simulink model "motorcontrol_19a_v2"  (R2019b)
settings: Solver=FixedStepDiscrete  StartTime=0.0  StopTime=Inf  FixedStep=Ts.pwm  MaxStep=5e-5  RelTol=1e-3  EnableMultiTasking=on
undefined symbols (not defined in the file): ControlMode, ctrlParams, dataType, DiscIntNeverNeededParam, Down, GPTRIP1SEL, GPTRIP2SEL, inverter, mcb_isSimVar, NumBits1, NumBits2, PI_params, pmsm, Slope1, Slope2, Target, Ts, TZ1, TZ2, Up
libraries: simulink x14, c2802xlib x7, c2837xDlib x3, c280xlib x1, c2000lib x1
(part 3 of 3)

== system motorcontrol_19a_v2/Motor_Control1/ControlSystem/Closed_Loop/Current_Controllers/FeedForward Decoupling Compensation ==
  d_current measured : Inport
  Electrical_speed measured : Inport  Port=2
  q_current measured : Inport  Port=3
  Add : Sum
  Constant : Constant  Value=pmsm.Ld  OutDataTypeStr=Inherit: Inherit via back propagation  SampleTime=-1
  Constant1 : Constant  Value=pmsm.FluxPM  OutDataTypeStr=Inherit: Inherit via back propagation  SampleTime=-1
  Constant2 : Constant  Value=pmsm.Lq  OutDataTypeStr=Inherit: Inherit via back propagation  SampleTime=-1
  Data Type Duplicate : DataTypeDuplicate  NumInputPorts=6
  Product4 : Product  Inputs=3
  Product5 : Product
  Product6 : Product
  Unary Minus : UnaryMinus
  q_voltage_compensation : Outport
  d_voltage_compensation : Outport  Port=2
  wires:
  q_current measured/1 -> Product4/2, Data Type Duplicate/1
  Constant1/1 -> Data Type Duplicate/5, Add/2
  Product6/1 -> d_voltage_compensation/1
  Product4/1 -> Unary Minus/1
  Unary Minus/1 -> q_voltage_compensation/1
  Constant/1 -> Data Type Duplicate/4, Product5/2
  Product5/1 -> Add/1
  Electrical_speed measured/1 -> Product4/3, Product6/1, Data Type Duplicate/2
  Add/1 -> Product6/2
  d_current measured/1 -> Product5/1, Data Type Duplicate/3
  Constant2/1 -> Product4/1, Data Type Duplicate/6

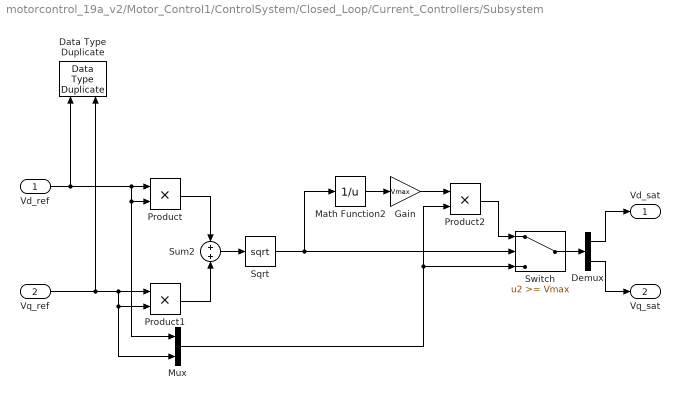
== system motorcontrol_19a_v2/Motor_Control1/ControlSystem/Closed_Loop/Current_Controllers/Subsystem ==
  Vd_ref : Inport
  Vq_ref : Inport  Port=2
  Data Type Duplicate : DataTypeDuplicate
  Demux : Demux  Outputs=2
  Gain : Gain  Gain=Vmax  OutDataTypeStr=Inherit: Same as input
  Math Function2 : Math  Operator=reciprocal  RndMeth=Simplest
  Mux : Mux  Inputs=2
  Product : Product  RndMeth=Simplest  OutDataTypeStr=Inherit: Same as first input
  Product1 : Product  RndMeth=Simplest  OutDataTypeStr=Inherit: Same as first input
  Product2 : Product  OutDataTypeStr=Inherit: Same as first input
  Sqrt : Sqrt  IntermediateResultsDataTypeStr=Inherit: Inherit from input  SaturateOnIntegerOverflow=on
  Sum2 : Sum  OutDataTypeStr=Inherit: Same as first input
  Switch : Switch  Threshold=Vmax  ZeroCross=off
  Vd_sat : Outport  VectorParamsAs1DForOutWhenUnconnected=off
  Vq_sat : Outport  Port=2  VectorParamsAs1DForOutWhenUnconnected=off
  wires:
  Vd_ref/1 -> Mux/1, Product/2, Product/1, Data Type Duplicate/1
  Demux/1 -> Vd_sat/1
  Product1/1 -> Sum2/2
  Product/1 -> Sum2/1
  Sum2/1 -> Sqrt/1
  Gain/1 -> Product2/1
  Math Function2/1 -> Gain/1
  Vq_ref/1 -> Mux/2, Product1/2, Product1/1, Data Type Duplicate/2
  Mux/1 -> Switch/3, Product2/2
  Product2/1 -> Switch/1
  Demux/2 -> Vq_sat/1
  Sqrt/1 -> Switch/2, Math Function2/1
  Switch/1 -> Demux/1

== system motorcontrol_19a_v2/Motor_Control1/ControlSystem/Closed_Loop/Sine-Cosine Lookup/Subsystem ==
  In1 : Inport
  Compare To Zero : simulink/Logic and Bit Operations/Compare To Zero  relop=<  OutDataTypeStr=boolean
  Data Type Conversion : DataTypeConversion  OutDataTypeStr=uint16  ConvertRealWorld=Stored Integer (SI)  RndMeth=Simplest
  If : If
  Merge : Merge
  Subsystem : Subsystem
  Subsystem1 : Subsystem
  convert_pu : Gain  Gain=1/(dlgSett.UpperSatLimit)  RndMeth=Simplest  OutDataTypeStr=Inherit: Same as input
  Out1 : Outport
  wires:
  If/2 -> Subsystem1/Action
  Subsystem/1(Out1) -> Merge/1
  convert_pu/1 -> Subsystem1/1(In1), Subsystem/1(In1), Compare To Zero/1
  In1/1 -> convert_pu/1
  If/1 -> Subsystem/Action
  Subsystem1/1(Out1) -> Merge/2
  Data Type Conversion/1 -> If/1
  Compare To Zero/1 -> Data Type Conversion/1
  Merge/1 -> Out1/1

== system motorcontrol_19a_v2/Motor_Control1/ControlSystem/Closed_Loop/Sine-Cosine Lookup/Subsystem1 ==
  In1 : Inport
  In2 : Inport  Port=2
  Demux : Demux
  Product : Product  RndMeth=Simplest  OutDataTypeStr=Inherit: Same as first input
  Product1 : Product  RndMeth=Simplest  OutDataTypeStr=Inherit: Same as first input
  Sum3 : Sum  Inputs=|+-  RndMeth=Simplest  OutDataTypeStr=Inherit: Same as first input
  Sum4 : Sum  Inputs=|++  RndMeth=Simplest  OutDataTypeStr=Inherit: Same as first input
  Sum5 : Sum  Inputs=|+-  RndMeth=Simplest  OutDataTypeStr=Inherit: Same as first input
  Sum6 : Sum  Inputs=|++  RndMeth=Simplest  OutDataTypeStr=Inherit: Same as first input
  Out1 : Outport
  Out2 : Outport  Port=2
  wires:
  Sum4/1 -> Out1/1
  Sum5/1 -> Product1/1
  Sum6/1 -> Out2/1
  Demux/1 -> Sum3/1
  Demux/2 -> Sum4/2, Sum3/2
  Product/1 -> Sum4/1
  Sum3/1 -> Product/1
  Product1/1 -> Sum6/1
  Demux/4 -> Sum5/2, Sum6/2
  In1/1 -> Demux/1
  Demux/3 -> Sum5/1
  In2/1 -> Product1/2, Product/2

== system motorcontrol_19a_v2/Motor_Control1/ControlSystem/Closed_Loop/Subsystem3/Subsystem ==
  d : Inport
  q : Inport  Port=2
  D_axis_aligned : Mux  Inputs=2
  Demux : Demux  Outputs=2
  Offset : Constant  Value=dlgSett.Offset  OutDataTypeStr=uint16  SampleTime=-1
  Q_axis_aligned : Mux  Inputs=2
  Switch : Switch  Criteria=u2 > Threshold  Threshold=1  RndMeth=Simplest  ZeroCross=off
  Unary_Minus : UnaryMinus
  d_axis : Outport  VectorParamsAs1DForOutWhenUnconnected=off
  q_axis : Outport  Port=2  VectorParamsAs1DForOutWhenUnconnected=off
  wires:
  d/1 -> D_axis_aligned/1, Q_axis_aligned/2
  Demux/1 -> d_axis/1
  Switch/1 -> Demux/1
  Offset/1 -> Switch/2
  D_axis_aligned/1 -> Switch/3
  q/1 -> D_axis_aligned/2, Unary_Minus/1
  Q_axis_aligned/1 -> Switch/1
  Demux/2 -> q_axis/1
  Unary_Minus/1 -> Q_axis_aligned/1

== system motorcontrol_19a_v2/Motor_Control1/ControlSystem/Closed_Loop/Subsystem4/Subsystem ==
  A : Inport
  B : Inport  Port=2
  D_axis_aligned : Mux  Inputs=2
  Demux : Demux  Outputs=2
  Offset : Constant  Value=dlgSett.Offset  OutDataTypeStr=uint16  SampleTime=-1
  Q_axis_aligned : Mux  Inputs=2
  Switch : Switch  Criteria=u2 > Threshold  Threshold=1  RndMeth=Simplest  ZeroCross=off
  Unary_Minus : UnaryMinus
  Alpha : Outport  VectorParamsAs1DForOutWhenUnconnected=off
  Beta : Outport  Port=2  VectorParamsAs1DForOutWhenUnconnected=off
  wires:
  Q_axis_aligned/1 -> Switch/1
  Demux/1 -> Alpha/1
  D_axis_aligned/1 -> Switch/3
  Switch/1 -> Demux/1
  A/1 -> Unary_Minus/1, D_axis_aligned/1
  Demux/2 -> Beta/1
  B/1 -> Q_axis_aligned/1, D_axis_aligned/2
  Offset/1 -> Switch/2
  Unary_Minus/1 -> Q_axis_aligned/2

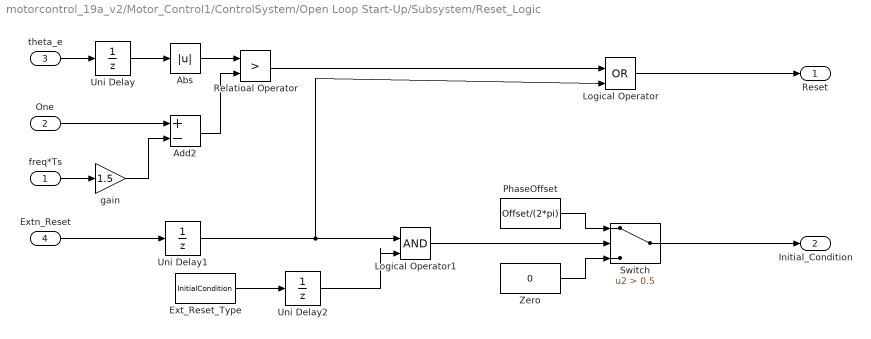
== system motorcontrol_19a_v2/Motor_Control1/ControlSystem/Open Loop Start-Up/Subsystem/Reset_Logic ==
  freq*Ts : Inport
  One : Inport  Port=2
  theta_e : Inport  Port=3
  Extn_Reset : Inport  Port=4
  Abs : Abs  RndMeth=Simplest
  Add2 : Sum  Inputs=+-  RndMeth=Simplest  OutDataTypeStr=Inherit: Same as first input
  Ext_Reset_Type : Constant  Value=InitialCondition  OutDataTypeStr=boolean  SampleTime=-1
  Logical Operator : Logic  Operator=OR  IconShape=distinctive  AllPortsSameDT=off  OutDataTypeStr=boolean
  Logical Operator1 : Logic  IconShape=distinctive  AllPortsSameDT=off  OutDataTypeStr=boolean
  PhaseOffset : Constant  Value=Offset/(2*pi)  OutDataTypeStr=Inherit: Inherit via back propagation  SampleTime=-1
  Relatioal Operator : RelationalOperator  Operator=>  OutDataTypeStr=boolean  RndMeth=Simplest  InputSameDT=on
  Switch : Switch  Criteria=u2 > Threshold  Threshold=0.5  OutDataTypeStr=Inherit: Inherit via back propagation  RndMeth=Simplest
  Uni Delay : UnitDelay  SampleTime=-1  HasFrameUpgradeWarning=on
  Uni Delay1 : UnitDelay  InitialCondition=1  SampleTime=-1  HasFrameUpgradeWarning=on
  Uni Delay2 : UnitDelay  InitialCondition=1  SampleTime=-1  HasFrameUpgradeWarning=on
  Zero : Constant  Value=0  OutDataTypeStr=Inherit: Inherit via back propagation  SampleTime=-1
  gain : Gain  Gain=1.5  RndMeth=Simplest  OutDataTypeStr=Inherit: Same as input
  Reset : Outport  VectorParamsAs1DForOutWhenUnconnected=off
  Initial_Condition : Outport  Port=2  VectorParamsAs1DForOutWhenUnconnected=off
  wires:
  Uni Delay2/1 -> Logical Operator1/2
  theta_e/1 -> Uni Delay/1
  gain/1 -> Add2/2
  Logical Operator1/1 -> Switch/2
  Ext_Reset_Type/1 -> Uni Delay2/1
  freq*Ts/1 -> gain/1
  Logical Operator/1 -> Reset/1
  Uni Delay/1 -> Abs/1
  One/1 -> Add2/1
  Switch/1 -> Initial_Condition/1
  Relatioal Operator/1 -> Logical Operator/1
  Uni Delay1/1 -> Logical Operator/2, Logical Operator1/1
  Extn_Reset/1 -> Uni Delay1/1
  Add2/1 -> Relatioal Operator/2
  Zero/1 -> Switch/3
  PhaseOffset/1 -> Switch/1
  Abs/1 -> Relatioal Operator/1

== system motorcontrol_19a_v2/Motor_Control1/ControlSystem/Open Loop Start-Up/Subsystem/Theta_IncrementSource ==
  In1 : Inport
  scale : Gain  Gain=1/(2*pi)  RndMeth=Simplest  OutDataTypeStr=Inherit: Same as input
  Out1 : Outport  VectorParamsAs1DForOutWhenUnconnected=off
  wires:
  In1/1 -> scale/1
  scale/1 -> Out1/1

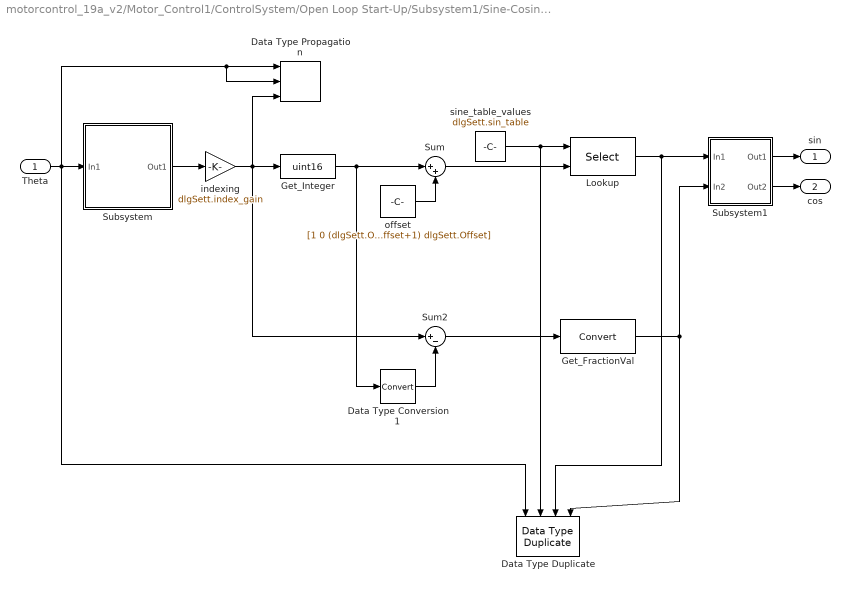
== system motorcontrol_19a_v2/Motor_Control1/ControlSystem/Open Loop Start-Up/Subsystem1/Sine-Cosine Lookup ==
  Theta : Inport
  Data Type Duplicate : DataTypeDuplicate  NumInputPorts=4
  Data Type Propagation : simulink/Signal Attributes/Data Type Propagation  PropDataType=fixdt(1, 16)  IfRefDouble=double  IfRefSingle=single  IsSigned=IsSigned1 or IsSigned2  NumBitsBase=max([NumBits1 NumBits2])  NumBitsMult=1  NumBitsAdd=0  NumBitsAllowFinal=1:128  PropScalingMode=Obtain via best precision  PropScaling=2^-10  ValuesUsedBestPrec=[0 dlgSett.index_gain]  SlopeBase=min([Slope1 Slope2])  SlopeMult=1  SlopeAdd=0  BiasBase=Bias1  BiasMult=1  BiasAdd=0
      settings: SourceProductName=Simulink  SourceProductBaseCode=SL
  Data Type Conversion1 : DataTypeConversion  RndMeth=Simplest
  Get_FractionVal : DataTypeConversion  RndMeth=Simplest
  Get_Integer : DataTypeConversion  OutDataTypeStr=uint16  RndMeth=Simplest
  Lookup : Selector  IndexMode=Zero-based  InputPortWidth=dlgSett.size  IndexOptions=Index vector (port)  Indices=[1 3]  OutputSizes=1
  Subsystem : Subsystem
  Subsystem1 : Subsystem
  Sum : Sum  Inputs=|++  AccumDataTypeStr=uint32  OutDataTypeStr=uint32  RndMeth=Simplest
  Sum2 : Sum  Inputs=|+-  RndMeth=Simplest  OutDataTypeStr=Inherit: Same as first input
  indexing : Gain  Gain=dlgSett.index_gain  OutDataTypeStr=Inherit: Inherit via back propagation  RndMeth=Simplest
  offset : Constant  Value=[1 0 (dlgSett.Offset+1) dlgSett.Offset]  OutDataTypeStr=int16  SampleTime=-1
  sine_table_values : Constant  Value=dlgSett.sin_table  OutDataTypeStr=Inherit: Inherit via back propagation  SampleTime=-1
  sin : Outport  VectorParamsAs1DForOutWhenUnconnected=off
  cos : Outport  Port=2  VectorParamsAs1DForOutWhenUnconnected=off
  wires:
  Subsystem1/2(Out2) -> cos/1
  Data Type Conversion1/1 -> Sum2/2
  Subsystem1/1(Out1) -> sin/1
  offset/1 -> Sum/2
  Lookup/1 -> Subsystem1/1(In1), Data Type Duplicate/3
  Get_FractionVal/1 -> Subsystem1/2(In2), Data Type Duplicate/4
  Sum/1 -> Lookup/2
  Theta/1 -> Subsystem/1(In1), Data Type Propagation/1, Data Type Propagation/2, Data Type Duplicate/1
  indexing/1 -> Get_Integer/1, Data Type Propagation/3, Sum2/1
  sine_table_values/1 -> Data Type Duplicate/2, Lookup/1
  Get_Integer/1 -> Data Type Conversion1/1, Sum/1
  Sum2/1 -> Get_FractionVal/1
  Subsystem/1(Out1) -> indexing/1

== system motorcontrol_19a_v2/Motor_Control1/ControlSystem/Open Loop Start-Up/Subsystem1/Subsystem1 ==
  In1 : Inport
  In2 : Inport  Port=2
  Data Type Duplicate : DataTypeDuplicate
  add_b : Sum  Inputs=-+  RndMeth=Simplest  OutDataTypeStr=Inherit: Same as first input
  add_c : Sum  Inputs=--  RndMeth=Simplest  OutDataTypeStr=Inherit: Same as first input
  one_by_two : Gain  Gain=1/2  RndMeth=Simplest  OutDataTypeStr=Inherit: Same as input
  sqrt3_by_two : Gain  Gain=sqrt(3)/2  RndMeth=Simplest  OutDataTypeStr=Inherit: Same as input
  a : Outport  VectorParamsAs1DForOutWhenUnconnected=off
  b : Outport  Port=2  VectorParamsAs1DForOutWhenUnconnected=off
  c : Outport  Port=3  VectorParamsAs1DForOutWhenUnconnected=off
  wires:
  add_c/1 -> c/1
  one_by_two/1 -> add_b/1, add_c/1
  In2/1 -> sqrt3_by_two/1, Data Type Duplicate/2
  sqrt3_by_two/1 -> add_c/2, add_b/2
  add_b/1 -> b/1
  In1/1 -> one_by_two/1, Data Type Duplicate/1, a/1

== system motorcontrol_19a_v2/Motor_Control1/ControlSystem/Open Loop Start-Up/Subsystem1/Subsystem2 ==
  Ds : Inport
  Qs : Inport  Port=2
  sin : Inport  Port=3
  cos : Inport  Port=4
  Data Type Duplicate : DataTypeDuplicate  NumInputPorts=4
  Subsystem : Subsystem
  dcos : Product  RndMeth=Simplest  OutDataTypeStr=Inherit: Same as first input
  dsin : Product  RndMeth=Simplest  OutDataTypeStr=Inherit: Same as first input
  qcos : Product  RndMeth=Simplest  OutDataTypeStr=Inherit: Same as first input
  qsin : Product  RndMeth=Simplest  OutDataTypeStr=Inherit: Same as first input
  sum_alpha : Sum  Inputs=|+-  RndMeth=Simplest  OutDataTypeStr=Inherit: Same as first input
  sum_beta : Sum  Inputs=|++  RndMeth=Simplest  OutDataTypeStr=Inherit: Same as first input
  Alpha : Outport  VectorParamsAs1DForOutWhenUnconnected=off
  Beta : Outport  Port=2  VectorParamsAs1DForOutWhenUnconnected=off
  wires:
  cos/1 -> qcos/2, dcos/2, Data Type Duplicate/3
  qsin/1 -> sum_alpha/2
  Subsystem/1(Alpha) -> Alpha/1
  Qs/1 -> qsin/1, qcos/1, Data Type Duplicate/2
  sum_beta/1 -> Subsystem/2(B)
  qcos/1 -> sum_beta/1
  dcos/1 -> sum_alpha/1
  Ds/1 -> dcos/1, dsin/1, Data Type Duplicate/1
  Subsystem/2(Beta) -> Beta/1
  sin/1 -> dsin/2, qsin/2, Data Type Duplicate/4
  sum_alpha/1 -> Subsystem/1(A)
  dsin/1 -> sum_beta/2

== system motorcontrol_19a_v2/Motor_Control1/Input Scaling/ Calculate Position and Speed/Subsystem2/PositionNoReset ==
  Index : Inport
  Count : Inport  Port=2
  Action Port : ActionPort
  CountsPerRevolution : Constant  Value=EncoderSlitsPerRevolution*4  OutDataTypeStr=Inherit: Inherit via back propagation
  MinMax : MinMax  Inputs=2  RndMeth=Simplest  ZeroCross=off
  Sum3 : Sum  Inputs=+-|  OutDataTypeStr=Inherit: Same as accumulator  RndMeth=Simplest
  Sum7 : Sum  Inputs=|++  OutDataTypeStr=Inherit: Same as accumulator  RndMeth=Simplest
  Position : Outport  VectorParamsAs1DForOutWhenUnconnected=off
  wires:
  Sum3/1 -> MinMax/1, Sum7/1
  Count/1 -> Sum3/1
  Index/1 -> Sum3/2
  CountsPerRevolution/1 -> Sum7/2
  Sum7/1 -> MinMax/2
  MinMax/1 -> Position/1

== system motorcontrol_19a_v2/Motor_Control1/Input Scaling/ Calculate Position and Speed/Subsystem2/PositionResetatIndex ==
  Count : Inport
  Action Port : ActionPort
  Position : Outport  VectorParamsAs1DForOutWhenUnconnected=off
  wires:
  Count/1 -> Position/1

== system motorcontrol_19a_v2/Motor_Control1/Input Scaling/ Calculate Position and Speed/Subsystem3/Subsystem ==
  ϴm : Inport
  In2 : Inport  Port=2
  If : If  NumInputs=2  IfExpression=u1 <= u2
  Merge : Merge
  Subsystem : Subsystem
  Subsystem1 : Subsystem
  Out1 : Outport
  wires:
  Merge/1 -> Out1/1
  If/2 -> Subsystem1/Action
  Subsystem/1(Out1) -> Merge/1
  ϴm/1 -> If/1, Subsystem/1(ϴm), Subsystem1/1(ϴm)
  If/1 -> Subsystem/Action
  Subsystem1/1(Out1) -> Merge/2
  In2/1 -> Subsystem/2(In2), Subsystem1/2(In2), If/2

== system motorcontrol_19a_v2/Motor_Control1/Input Scaling/ Calculate Position and Speed/Subsystem3/Subsystem1 ==
  In1 : Inport
  Add : Sum  Inputs=-+  OutDataTypeStr=Inherit: Inherit via back propagation  RndMeth=Simplest
  Floor : Rounding
  Multiply : Gain  Gain=1/maxAngleIn  RndMeth=Simplest  OutDataTypeStr=Inherit: Same as input
  Multiply1 : Gain  Gain=maxAngleIn  OutDataTypeStr=Inherit: Inherit via back propagation  RndMeth=Simplest
  Number of pole pairs : Gain  Gain=NrPP  RndMeth=Simplest  OutDataTypeStr=Inherit: Same as input
  Out1 : Outport
  ϴe : Outport  Port=2
  wires:
  Multiply1/1 -> Add/1
  Number of pole pairs/1 -> Multiply/1, Add/2
  Add/1 -> ϴe/1, Out1/1
  Floor/1 -> Multiply1/1
  Multiply/1 -> Floor/1
  In1/1 -> Number of pole pairs/1

== system motorcontrol_19a_v2/Motor_Control1/ControlSystem/Closed_Loop/Sine-Cosine Lookup/Subsystem/Subsystem ==
  In1 : Inport
  Action Port : ActionPort
  Convert_back : DataTypeConversion  RndMeth=Simplest
  Convert_uint16 : DataTypeConversion  OutDataTypeStr=int16
  Data Type Duplicate : DataTypeDuplicate
  Sum : Sum  Inputs=|+-  RndMeth=Simplest  OutDataTypeStr=Inherit: Same as first input
  Out1 : Outport
  wires:
  In1/1 -> Data Type Duplicate/1, Sum/1, Convert_uint16/1
  Convert_uint16/1 -> Convert_back/1
  Convert_back/1 -> Sum/2, Data Type Duplicate/2
  Sum/1 -> Out1/1

== system motorcontrol_19a_v2/Motor_Control1/ControlSystem/Closed_Loop/Sine-Cosine Lookup/Subsystem/Subsystem1 ==
  In1 : Inport
  Action Port : ActionPort
  Convert_back : DataTypeConversion  RndMeth=Simplest
  Convert_uint16 : DataTypeConversion  OutDataTypeStr=int16  RndMeth=Simplest
  Data Type Duplicate : DataTypeDuplicate
  Sum : Sum  Inputs=|+-  RndMeth=Simplest  OutDataTypeStr=Inherit: Same as first input
  Out1 : Outport
  wires:
  Convert_uint16/1 -> Convert_back/1
  In1/1 -> Data Type Duplicate/1, Sum/1, Convert_uint16/1
  Convert_back/1 -> Sum/2, Data Type Duplicate/2
  Sum/1 -> Out1/1

== system motorcontrol_19a_v2/Motor_Control1/ControlSystem/Open Loop Start-Up/Subsystem1/Sine-Cosine Lookup/Subsystem ==
  In1 : Inport
  Compare To Zero : simulink/Logic and Bit Operations/Compare To Zero  relop=<  OutDataTypeStr=boolean
  Data Type Conversion : DataTypeConversion  OutDataTypeStr=uint16  ConvertRealWorld=Stored Integer (SI)  RndMeth=Simplest
  If : If
  Merge : Merge
  Subsystem : Subsystem
  Subsystem1 : Subsystem
  convert_pu : Gain  Gain=1/(dlgSett.UpperSatLimit)  RndMeth=Simplest  OutDataTypeStr=Inherit: Same as input
  Out1 : Outport
  wires:
  If/2 -> Subsystem1/Action
  Subsystem/1(Out1) -> Merge/1
  convert_pu/1 -> Subsystem1/1(In1), Subsystem/1(In1), Compare To Zero/1
  In1/1 -> convert_pu/1
  If/1 -> Subsystem/Action
  Subsystem1/1(Out1) -> Merge/2
  Data Type Conversion/1 -> If/1
  Compare To Zero/1 -> Data Type Conversion/1
  Merge/1 -> Out1/1

== system motorcontrol_19a_v2/Motor_Control1/ControlSystem/Open Loop Start-Up/Subsystem1/Sine-Cosine Lookup/Subsystem1 ==
  In1 : Inport
  In2 : Inport  Port=2
  Demux : Demux
  Product : Product  RndMeth=Simplest  OutDataTypeStr=Inherit: Same as first input
  Product1 : Product  RndMeth=Simplest  OutDataTypeStr=Inherit: Same as first input
  Sum3 : Sum  Inputs=|+-  RndMeth=Simplest  OutDataTypeStr=Inherit: Same as first input
  Sum4 : Sum  Inputs=|++  RndMeth=Simplest  OutDataTypeStr=Inherit: Same as first input
  Sum5 : Sum  Inputs=|+-  RndMeth=Simplest  OutDataTypeStr=Inherit: Same as first input
  Sum6 : Sum  Inputs=|++  RndMeth=Simplest  OutDataTypeStr=Inherit: Same as first input
  Out1 : Outport
  Out2 : Outport  Port=2
  wires:
  Sum4/1 -> Out1/1
  Sum5/1 -> Product1/1
  Sum6/1 -> Out2/1
  Demux/1 -> Sum3/1
  Demux/2 -> Sum4/2, Sum3/2
  Product/1 -> Sum4/1
  Sum3/1 -> Product/1
  Product1/1 -> Sum6/1
  Demux/4 -> Sum5/2, Sum6/2
  In1/1 -> Demux/1
  Demux/3 -> Sum5/1
  In2/1 -> Product1/2, Product/2

== system motorcontrol_19a_v2/Motor_Control1/ControlSystem/Open Loop Start-Up/Subsystem1/Subsystem2/Subsystem ==
  A : Inport
  B : Inport  Port=2
  D_axis_aligned : Mux  Inputs=2
  Demux : Demux  Outputs=2
  Offset : Constant  Value=dlgSett.Offset  OutDataTypeStr=uint16  SampleTime=-1
  Q_axis_aligned : Mux  Inputs=2
  Switch : Switch  Criteria=u2 > Threshold  Threshold=1  RndMeth=Simplest  ZeroCross=off
  Unary_Minus : UnaryMinus
  Alpha : Outport  VectorParamsAs1DForOutWhenUnconnected=off
  Beta : Outport  Port=2  VectorParamsAs1DForOutWhenUnconnected=off
  wires:
  Unary_Minus/1 -> Q_axis_aligned/2
  Offset/1 -> Switch/2
  B/1 -> D_axis_aligned/2, Q_axis_aligned/1
  Demux/2 -> Beta/1
  A/1 -> D_axis_aligned/1, Unary_Minus/1
  Switch/1 -> Demux/1
  D_axis_aligned/1 -> Switch/3
  Demux/1 -> Alpha/1
  Q_axis_aligned/1 -> Switch/1

== system motorcontrol_19a_v2/Motor_Control1/Input Scaling/ Calculate Position and Speed/Subsystem3/Subsystem/Subsystem ==
  ϴm : Inport
  In2 : Inport  Port=2
  Action Port : ActionPort
  Add : Sum  Inputs=++-  RndMeth=Simplest  OutDataTypeStr=Inherit: Same as first input
  Constant : Constant  Value=maxAngleIn  OutDataTypeStr=Inherit: Inherit via back propagation
  Out1 : Outport
  wires:
  Add/1 -> Out1/1
  ϴm/1 -> Add/1
  Constant/1 -> Add/2
  In2/1 -> Add/3

== system motorcontrol_19a_v2/Motor_Control1/Input Scaling/ Calculate Position and Speed/Subsystem3/Subsystem/Subsystem1 ==
  ϴm : Inport
  In2 : Inport  Port=2
  Action Port : ActionPort
  Add : Sum  Inputs=+-  RndMeth=Simplest  OutDataTypeStr=Inherit: Same as first input
  Out1 : Outport
  wires:
  Add/1 -> Out1/1
  ϴm/1 -> Add/1
  In2/1 -> Add/2

== system motorcontrol_19a_v2/Motor_Control1/ControlSystem/Open Loop Start-Up/Subsystem1/Sine-Cosine Lookup/Subsystem/Subsystem ==
  In1 : Inport
  Action Port : ActionPort
  Convert_back : DataTypeConversion  RndMeth=Simplest
  Convert_uint16 : DataTypeConversion  OutDataTypeStr=int16
  Data Type Duplicate : DataTypeDuplicate
  Sum : Sum  Inputs=|+-  RndMeth=Simplest  OutDataTypeStr=Inherit: Same as first input
  Out1 : Outport
  wires:
  In1/1 -> Data Type Duplicate/1, Sum/1, Convert_uint16/1
  Convert_uint16/1 -> Convert_back/1
  Convert_back/1 -> Sum/2, Data Type Duplicate/2
  Sum/1 -> Out1/1

== system motorcontrol_19a_v2/Motor_Control1/ControlSystem/Open Loop Start-Up/Subsystem1/Sine-Cosine Lookup/Subsystem/Subsystem1 ==
  In1 : Inport
  Action Port : ActionPort
  Convert_back : DataTypeConversion  RndMeth=Simplest
  Convert_uint16 : DataTypeConversion  OutDataTypeStr=int16  RndMeth=Simplest
  Data Type Duplicate : DataTypeDuplicate
  Sum : Sum  Inputs=|+-  RndMeth=Simplest  OutDataTypeStr=Inherit: Same as first input
  Out1 : Outport
  wires:
  Convert_uint16/1 -> Convert_back/1
  In1/1 -> Data Type Duplicate/1, Sum/1, Convert_uint16/1
  Convert_back/1 -> Sum/2, Data Type Duplicate/2
  Sum/1 -> Out1/1

== stateflow chart motorcontrol_19a_v2/Mode_Scheduler/Controller_Mode_Scheduler ==
  settings: updateMethod=DISCRETE  executeAtInitialization=1
  note: Controller Mode Scheduler
  note: The motor control algorithm begins in a stand-by mode awaiting a command to turn the motor on. Once this command
      | is issued the motor rotates to identify a known rotor position with valid position. The appropriate closed loop control then begins.
      | Upon a request to stop the motor, the motor will decellerate until zero speed is identified, after which the algorithm returns to the stand-by mode.
  state Stand_By
    entry: controller_mode = SpeedControl;
    velocity_command=0;
    torque_command = 0;
  state Motor_On
    state Motor_Control
      state Speed_Control
        entry: controller_mode = SpeedControl;
        en, du:
        velocity_command = command;
      state Position_Control
        entry: controller_mode = PositionControl;
        en,du:
        position_command = command;
      state Torque_Control
        entry: controller_mode = TorqueControl;
        en, du:
        torque_command = command;
      (default) -> (junction 386)
      (junction 386) -> Speed_Control [order 1] : [command_type==Speed]
      (junction 386) -> (junction 387) [order 2]
      (junction 387) -> Position_Control [order 1] : [command_type==Position]
      (junction 387) -> (junction 388) [order 2]
      (junction 388) -> Torque_Control : % [command_type==Torque]
  (default) -> Stand_By
  Stand_By -> Motor_On : [motor_on]
  Motor_On -> Stand_By : [~motor_on]
  data: controller_mode output Enum: ControllerMode; velocity_command output dataType; motor_on input boolean; position_command output dataType; command_type input Enum: ControlMode; torque_command output dataType; command input dataType
